simulink model "Simulink_Project1"  (R2023b)
settings: Solver=VariableStepAuto  StartTime=0.0  StopTime=168  RelTol=1e-3
values from neighbouring files (symbols this model uses):
  F1 = 10.0    (= 10)    [Call.m]    (also in Callplot.m; S_fun_sep.m = u(5); nonlinearcon.m)
  F2 = xOpt(6)    [Call.m]    (also in Callplot.m; S_fun_sep.m = u(1); minCostFunction.m = x(6); nonlinearcon.m = x(6))
  F200 = xOpt(2)    [Call.m]    (also in Callplot.m; S_fun_sep.m = u(4); minCostFunction.m = x(2); nonlinearcon.m = x(2))
  F3 = xOpt(5)    [Call.m]    (also in Callplot.m; S_fun_sep.m = u(2); minCostFunction.m = x(5); nonlinearcon.m = x(5))
  L2 = xOpt(7)    [Call.m]    (also in Callplot.m; S_fun_sep.m = x(1); minCostFunction.m = x(2); nonlinearcon.m = x(7))
  P100 = xOpt(4)    [Call.m]    (also in Callplot.m; S_fun_sep.m = u(3); minCostFunction.m = x(4); nonlinearcon.m = 194.7)
  T1 = 40.0    (= 40)    [Call.m]    (also in Callplot.m; S_fun_sep.m = u(7); nonlinearcon.m)
  T200 = 25.0    (= 25)    [Call.m]    (also in Callplot.m; S_fun_sep.m = u(8); nonlinearcon.m)
  X1 = 5.0    (= 5)    [Call.m]    (also in Callplot.m; S_fun_sep.m = u(6); nonlinearcon.m)
libraries: slpidlib x1
settings Model: Creator=bjark  LastModifiedBy=bjark

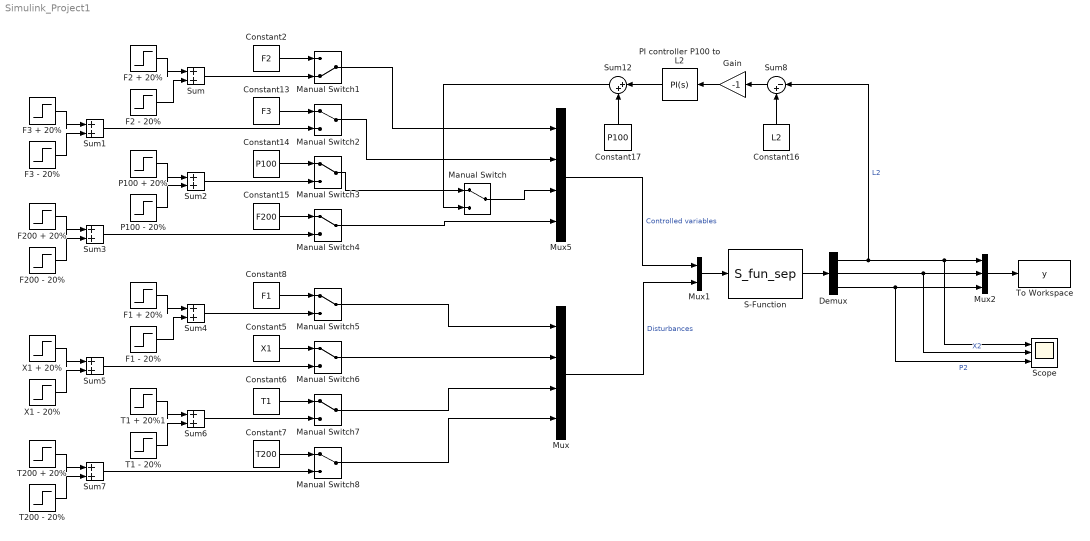
== system Simulink_Project1 ==
  Constant13 : Constant  Value=F3
  Constant14 : Constant  Value=P100
  Constant15 : Constant  Value=F200
  Constant16 : Constant  Value=L2
  Constant17 : Constant  Value=P100
  Constant2 : Constant  Value=F2
  Constant5 : Constant  Value=X1
  Constant6 : Constant  Value=T1
  Constant7 : Constant  Value=T200
  Constant8 : Constant  Value=F1
  Demux : Demux  Outputs=3
  F1 + 20% : Step  Time=10  Before=F1  After=F1+(F1*0.2)  SampleTime=0
  F1 - 20% : Step  Time=60  After=-(F1*0.2)  SampleTime=0
  F2 + 20% : Step  Time=10  Before=F2  After=F2+(F2*0.2)  SampleTime=0
  F2 - 20% : Step  Time=60  After=-(F2*0.2)  SampleTime=0
  F200 + 20% : Step  Time=10  Before=F200  After=F200+(F200*0.2)  SampleTime=0
  F200 - 20% : Step  Time=60  After=-(F200*0.2)  SampleTime=0
  F3 + 20% : Step  Time=10  Before=F3  After=F3+(F3*0.2)  SampleTime=0
  F3 - 20% : Step  Time=60  After=-(F3*0.2)  SampleTime=0
  Gain : Gain  Gain=-1
  Manual Switch{,2..8} (8 alike) : ManualSwitch
  Manual Switch1 : ManualSwitch  CurrentSetting=0
  Mux : Mux
  Mux1 : Mux  Inputs=2
  Mux2 : Mux  Inputs=3
  Mux5 : Mux
  P100 + 20% : Step  Time=10  Before=P100  After=P100+(P100*0.2)  SampleTime=0
  P100 - 20% : Step  Time=60  After=-(P100*0.2)  SampleTime=0
  PI controller P100 to L2 : slpidlib/PID Controller  Controller=PI  Form=Parallel  TimeDomain=Continuous-time  UseExternalTs=off  SampleTime=-1  IntegratorMethod=Forward Euler  FilterMethod=Forward Euler  ControllerParametersSource=internal  P=400  I=0.5  UseKiTs=off  D=0  N=100  UseFilter=on  TunerSelectOption=Transfer Function Based (PID Tuner App)  InitialConditionSource=internal  InitialConditionForIntegrator=0  InitialConditionForFilter=0  DifferentiatorICPrevScaledInput=0  ExternalReset=none  TrackingMode=off  Kt=1  LimitOutput=off  SatLimitsSource=internal  UpperSaturationLimit=inf  LowerSaturationLimit=-inf  LinearizeAsGain=on  AntiWindupMode=none  Kb=1  LimitIntegrator=off  UpperIntegratorSaturationLimit=inf  LowerIntegratorSaturationLimit=-inf  POutMin=[]  POutMax=[]  IOutMin=[]  IOutMax=[]  DOutMin=[]  DOutMax=[]  NOutMin=[]  NOutMax=[]  SumOutMin=[]  SumOutMax=[]  SaturationOutMin=[]  SaturationOutMax=[]  PParamMin=[]  PParamMax=[]  IParamMin=[]  IParamMax=[]  DParamMin=[]  DParamMax=[]  NParamMin=[]  NParamMax=[]  KbParamMin=[]  KbParamMax=[]  KtParamMin=[]  KtParamMax=[]  KbOutMin=[]  KbOutMax=[]  KtOutMin=[]  KtOutMax=[]  IntegratorOutMin=[]  IntegratorOutMax=[]  FilterOutMin=[]  FilterOutMax=[]  SumI1OutMin=[]  SumI1OutMax=[]  SumI2OutMin=[]  SumI2OutMax=[]  SumI3OutMin=[]  SumI3OutMax=[]  SumI4OutMin=[]  SumI4OutMax=[]  SumDOutMin=[]  SumDOutMax=[]  DifferentiatorOutMin=[]  DifferentiatorOutMax=[]  FilterDiffOutCoefMin=[]  FilterDiffOutCoefMax=[]  ReciprocalOutMin=[]  ReciprocalOutMax=[]  SumDenOutMin=[]  SumDenOutMax=[]  SumNumOutMin=[]  SumNumOutMax=[]  DivideOutMin=[]  DivideOutMax=[]  UdiffTsProdOutMin=[]  UdiffTsProdOutMax=[]  NTsProdOutMin=[]  NTsProdOutMax=[]  UintegralTsProdOutMin=[]  UintegralTsProdOutMax=[]  UngainTsProdOutMin=[]  UngainTsProdOutMax=[]  ClampingZeroOutDataTypeStr=Inherit: Inherit via back propagation  ClampingZeroOutMin=[]  ClampingZeroOutMax=[]  FilterDenConstantOutDataTypeStr=Inherit: Inherit via back propagation  FilterDenConstantOutMin=[]  FilterDenConstantOutMax=[]  PCopyOutDataTypeStr=Inherit: Inherit via back propagation  PCopyOutMin=[]  PCopyOutMax=[]  NCopyOutDataTypeStr=Inherit: Inherit via back propagation  NCopyOutMin=[]  NCopyOutMax=[]  IntegratorContinuousStateAttributes=''  IntegratorStateMustResolveToSignalObject=off  IntegratorRTWStateStorageClass=Auto  FilterContinuousStateAttributes=''  FilterStateMustResolveToSignalObject=off  FilterRTWStateStorageClass=Auto  ParallelPVariant=InternalParameters  IdealPVariant=Disabled  IVariant=InternalParameters  DVariant=Disabled  IntegratorVariant=Continuous  SatVariant=Disabled  AWVariant=Passthrough  PCopyVariant=Disabled  TRVariant=Disabled  FdbkBlocksVariant=Forward  IdealPFdbkVariant=Disabled  SatFdbkVariant=Disabled  DerivativeFilterVariant=Disabled  NVariant=Disabled  NCopyVariant=Disabled_SignalSpec  FilterICVariant=Disabled  IntegratorICVariant=InternalICs  ExternalResetVariant=Disabled  TRSumVariant=Passthrough  SumFdbkVariant=Disabled  SumVariant=Sum_PI  TsampFilterVariant=InternalTs  TsampNgainVariant=Passthrough  TsampIntegralVariant=Disabled_SignalSpec  ExternalSaturationOutDataTypeStr=Inherit: Same as second input
  S-Function : S-Function  FunctionName=S_fun_sep  Parameters=xinit, par  SFunctionDeploymentMode=off  EnableBusSupport=off
  Scope : Scope  NumInputPorts=3
  Sum{,1..7,12} (9 alike) : Sum  Inputs=|++
  Sum8 : Sum  Inputs=|-+
  T1 + 20%1 : Step  Time=10  Before=T1  After=T1+(F2*0.2)  SampleTime=0
  T1 - 20% : Step  Time=60  After=-(T1*0.2)  SampleTime=0
  T200 + 20% : Step  Time=10  Before=T200  After=T200+(T200*0.2)  SampleTime=0
  T200 - 20% : Step  Time=60  After=-(T200*0.2)  SampleTime=0
  To Workspace : ToWorkspace  VariableName=y  SampleTime=-1
  X1 + 20% : Step  Time=10  Before=X1  After=X1+(X1*0.2)  SampleTime=0
  X1 - 20% : Step  Time=60  After=-(X1*0.2)  SampleTime=0
  wires:
  Mux1/1 -> S-Function/1
  S-Function/1 -> Demux/1
  Mux2/1 -> To Workspace/1
  Demux/2 -> Scope/2, Mux2/2  "X2"
  Demux/3 -> Scope/3, Mux2/3  "P2"
  Demux/1 -> Sum8/1, Scope/1, Mux2/1  "L2"
  Mux5/1 -> Mux1/1  "Controlled variables"
  Mux/1 -> Mux1/2  "Disturbances"
  Constant16/1 -> Sum8/2
  PI controller P100 to L2/1 -> Sum12/1
  Constant17/1 -> Sum12/2
  Manual Switch/1 -> Mux5/3
  Sum12/1 -> Manual Switch/2
  Constant2/1 -> Manual Switch1/1
  Manual Switch1/1 -> Mux5/1
  Constant13/1 -> Manual Switch2/1
  Manual Switch2/1 -> Mux5/2
  Constant14/1 -> Manual Switch3/1
  Manual Switch3/1 -> Manual Switch/1
  Constant15/1 -> Manual Switch4/1
  Manual Switch4/1 -> Mux5/4
  F2 + 20%/1 -> Sum/1
  F2 - 20%/1 -> Sum/2
  Sum/1 -> Manual Switch1/2
  F3 + 20%/1 -> Sum1/1
  F3 - 20%/1 -> Sum1/2
  Sum1/1 -> Manual Switch2/2
  P100 + 20%/1 -> Sum2/1
  P100 - 20%/1 -> Sum2/2
  Sum2/1 -> Manual Switch3/2
  F200 + 20%/1 -> Sum3/1
  F200 - 20%/1 -> Sum3/2
  Sum3/1 -> Manual Switch4/2
  T200 - 20%/1 -> Sum7/2
  T200 + 20%/1 -> Sum7/1
  Sum7/1 -> Manual Switch8/2
  Sum5/1 -> Manual Switch6/2
  F1 + 20%/1 -> Sum4/1
  T1 - 20%/1 -> Sum6/2
  Constant6/1 -> Manual Switch7/1
  X1 - 20%/1 -> Sum5/2
  T1 + 20%1/1 -> Sum6/1
  Sum6/1 -> Manual Switch7/2
  X1 + 20%/1 -> Sum5/1
  Constant7/1 -> Manual Switch8/1
  F1 - 20%/1 -> Sum4/2
  Sum4/1 -> Manual Switch5/2
  Constant5/1 -> Manual Switch6/1
  Constant8/1 -> Manual Switch5/1
  Manual Switch5/1 -> Mux/1
  Manual Switch6/1 -> Mux/2
  Manual Switch7/1 -> Mux/3
  Manual Switch8/1 -> Mux/4
  Gain/1 -> PI controller P100 to L2/1
  Sum8/1 -> Gain/1
